simulink model "test_update"  (R2023b)
settings: Solver=VariableStepAuto  StartTime=0.0  StopTime=6  RelTol=1e-3
libraries: sensors_subsystems x1
settings Model: Creator=brent  LastModifiedBy=brent

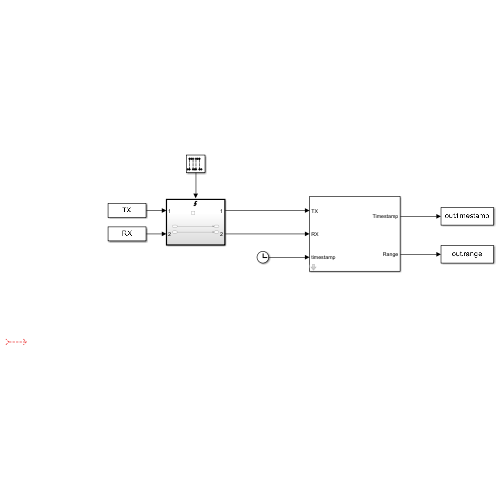
[thumbnail: Simulink's stored preview of the top-level diagram]
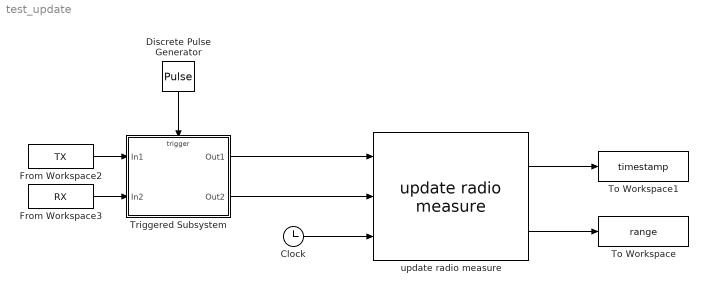
== system test_update ==
  Clock : Clock
  Discrete Pulse Generator : DiscretePulseGenerator  Period=10  SampleTime=0.1
  From Workspace2 : FromWorkspace  VariableName=TX
  From Workspace3 : FromWorkspace  VariableName=RX
  To Workspace : ToWorkspace  VariableName=range  SaveFormat=Timeseries  SampleTime=-1
  To Workspace1 : ToWorkspace  VariableName=timestamp  SaveFormat=Timeseries  SampleTime=-1
  Triggered Subsystem : Subsystem  TreatAsAtomicUnit=on
  update radio measure : sensors_subsystems/update radio measure  R_m=R_M
      settings: SourceProductName=Sensors library
  wires:
  Clock/1 -> update radio measure/3
  update radio measure/1 -> To Workspace1/1
  From Workspace2/1 -> Triggered Subsystem/1(In1)
  Discrete Pulse Generator/1 -> Triggered Subsystem/Trigger
  Triggered Subsystem/1(Out1) -> update radio measure/1
  ? -> ?
  From Workspace3/1 -> Triggered Subsystem/2(In2)
  Triggered Subsystem/2(Out2) -> update radio measure/2
  update radio measure/2 -> To Workspace/1

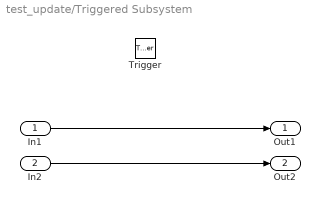
== system test_update/Triggered Subsystem ==
  In1 : Inport
  In2 : Inport  Port=2
  Trigger : TriggerPort  VariantControl=(inherit)
  Out1 : Outport
  Out2 : Outport  Port=2
  wires:
  In1/1 -> Out1/1
  In2/1 -> Out2/1
